simulink model "PEMFuelCellSystem_GasMixture_cEGR_RouteA_v2_v01"  (R2025b)
settings: Solver=VariableStepAuto  StartTime=0.0  StopTime=2500  RelTol=1e-3  AbsTol=1e-3
model workspace: external: MATLAB File E:\agentwork_pemfc_cEGR_0519\04_Simulink物理网络模型\01_模型\RouteA_GasMixture_Derived\PEMFuelCellSystemWithACustomLibraryParameters.m (data not in the file)
undefined symbols (not defined in the file): anode_tube_D, cathode_tube_D, cegr_valve_max_area, cegr_valve_open_min_area, comp_rpm_TLU, coolant_num_layers, coolant_num_passes, coolant_tube_D, coolant_w_channels, env_p, env_T, env_yH20, env_yO2, radiator_air_area_fins, radiator_air_area_primary, radiator_eta_fin, radiator_N_tubes, radiator_rho, radiator_t_wall, radiator_tube_H, radiator_W, routeA_air_pid_Ki, routeA_air_pid_Kp, routeA_anode_source_conditioner_nominal_flow_kg_s, routeA_cathode_source_conditioner_nominal_flow_kg_s, routeA_egr_control_Ki_area, routeA_egr_control_Kp_area, routeA_egr_target_input_mode_id, routeA_egr_valve_actuator_tau, routeA_egr_valve_area_direct, routeA_target_egr_ratio_comp_in, routeA_voltage_current_max_A, routeA_voltage_current_min_A, routeA_voltage_pi_Ki, routeA_voltage_pi_Kp, stack_area, stack_iL, stack_mea_rho, stack_num_cells, stack_num_channels, stack_t_gdl, stack_t_membrane, stack_w_channels, tank_p, tank_T, tank_yH2
libraries: FuelCell_lib x67, fl_lib x67, nesl_utility x56, slpidlib x5
(part 3 of 6)

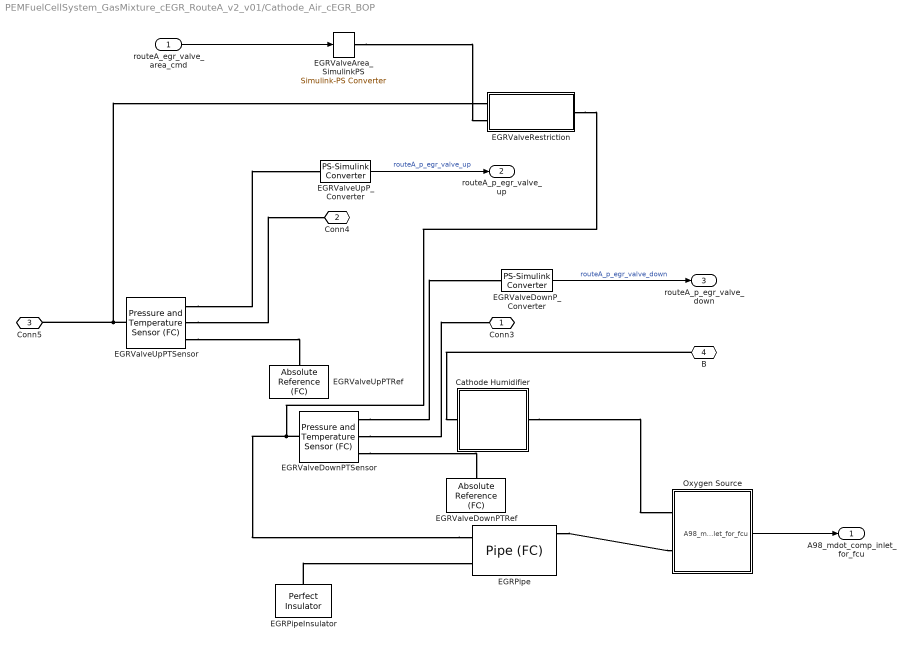
== system PEMFuelCellSystem_GasMixture_cEGR_RouteA_v2_v01/Cathode_Air_cEGR_BOP ==
  routeA_egr_valve_area_cmd : Inport
  Cathode Humidifier : Subsystem  Tag=PublishSubsystem
  EGRPipe : FuelCell_lib/elements/Pipe (FC)  length=cegr_pipe_length m  area=cegr_pipe_area m^2  Dh=cegr_pipe_D m  extra_length=cegr_pipe_extra_length m  roughness=cegr_pipe_roughness m  Re_lam=2000  Re_tur=4000  shape_factor=64  Nu_lam=3.66  tau_c=cegr_cond_tau s  isCond=[0; 0; 0; 1]  volMeas=false  compMeas=FuelCell.enum.Composition.Mole  p0=cegr_pipe_p0 MPa  T0=env_T degC  comp=FuelCell.enum.Composition.Mole  y0=[1-env_yO2-env_yH20; env_yO2; 0; env_yH20]  x0=[1-env_yO2-env_yH20; env_yO2; 0; env_yH20]
      settings: InternalSimscapePortConfiguration="{\"Bottom\":[{\"id\":\"MIn\",\"label\":\"M_in\",\"type\":\"input\"},{\"id\":\"TIn\",\"label\":\"T_in\",\"type\":\"input\"}],\"Left\":[{\"id\":\"A\",\"label\":\"A\",\"type\":\"FuelCell.FuelCell\"},{\"id\":\"H\",\"label\":\"H\",\"type\":\"foundation.thermal.thermal\"}],\"Right\":[{\"id\":\"B\",\"label\":\"B\",\"type\":\"FuelCell.FuelCell\"}],\"Top\":[]}"
  EGRPipeInsulator : fl_lib/Thermal/Thermal Elements/Perfect Insulator  T_specify=off  T_priority=None  T=293.15 K  T_nominal_specify=off  T_nominal_value=1  T_nominal_unit=K
  EGRValveArea_SimulinkPS : nesl_utility/Simulink-PS Converter  PhysicalDomain=network_engine_domain  SubClassName=ps_input  LeftPortType=input  RightPortType=output  PseudoPeriodic=off  Frequencies=[]  NoiseDistribution=none  NoiseParameters=[]  Unit=m^2  AffineConversion=off  FilteringAndDerivatives=provide  SimscapeFilterOrder=1  InputFilterTimeConstant=0.001  UdotUserProvided=0
  EGRValveDownPTRef : FuelCell_lib/elements/Absolute Reference (FC)
      settings: InternalSimscapePortConfiguration="{\"Bottom\":[],\"Left\":[{\"id\":\"A\",\"label\":\"\",\"type\":\"FuelCell.FuelCell\"}],\"Right\":[],\"Top\":[]}"
  EGRValveDownPTSensor : FuelCell_lib/sensors/Pressure and Temperature Sensor (FC)
      settings: InternalSimscapePortConfiguration="{\"Bottom\":[],\"Left\":[{\"id\":\"A\",\"label\":\"A\",\"type\":\"FuelCell.FuelCell\"}],\"Right\":[{\"id\":\"P\",\"label\":\"P\",\"type\":\"output\"},{\"id\":\"T\",\"label\":\"T\",\"type\":\"output\"},{\"id\":\"B\",\"label\":\"B\",\"type\":\"FuelCell.FuelCell\"}],\"Top\":[]}"
  EGRValveDownP_Converter : nesl_utility/PS-Simulink Converter  PhysicalDomain=network_engine_domain  SubClassName=ps_output  LeftPortType=input  RightPortType=output  PseudoPeriodic=off  Frequencies=[]  VectorFormat=inherit  Unit=inherit  AffineConversion=off
  EGRValveRestriction : Subsystem  Variant=on
  EGRValveUpPTRef : FuelCell_lib/elements/Absolute Reference (FC)
      settings: InternalSimscapePortConfiguration="{\"Bottom\":[],\"Left\":[{\"id\":\"A\",\"label\":\"\",\"type\":\"FuelCell.FuelCell\"}],\"Right\":[],\"Top\":[]}"
  EGRValveUpPTSensor : FuelCell_lib/sensors/Pressure and Temperature Sensor (FC)
      settings: InternalSimscapePortConfiguration="{\"Bottom\":[],\"Left\":[{\"id\":\"A\",\"label\":\"A\",\"type\":\"FuelCell.FuelCell\"}],\"Right\":[{\"id\":\"P\",\"label\":\"P\",\"type\":\"output\"},{\"id\":\"T\",\"label\":\"T\",\"type\":\"output\"},{\"id\":\"B\",\"label\":\"B\",\"type\":\"FuelCell.FuelCell\"}],\"Top\":[]}"
  EGRValveUpP_Converter : nesl_utility/PS-Simulink Converter  PhysicalDomain=network_engine_domain  SubClassName=ps_output  LeftPortType=input  RightPortType=output  PseudoPeriodic=off  Frequencies=[]  VectorFormat=inherit  Unit=inherit  AffineConversion=off
  Oxygen Source : Subsystem  Tag=PublishSubsystem
      mask Display:
      | plot(0, 0)
      | plot(100, 100)
      | 
      | n = 80;
      | r1 = 15;
      | r2 = 30;
      | 
      | plot(cos(linspace(0, 2*pi, n))*r1 + 65, sin(linspace(0, 2*pi, n))*r1 + 50)
      | plot(cos(linspace(0, 2*pi, n))*r2 + 65, sin(linspace(0, 2*pi, n))*r2 + 50)
      | 
      | plot([65 30 30 42], [80 80 70 70])
  Conn3 : PMIOPort  Side=Right
  Conn4 : PMIOPort  Port=2  Side=Right
  Conn5 : PMIOPort  Port=3  Side=Left
  B : PMIOPort  Port=4  Side=Left
  A98_mdot_comp_inlet_for_fcu : Outport
  routeA_p_egr_valve_up : Outport  Port=2
  routeA_p_egr_valve_down : Outport  Port=3
  wires:
  routeA_egr_valve_area_cmd/1 -> EGRValveArea_SimulinkPS/1
  EGRValveUpP_Converter/1 -> routeA_p_egr_valve_up/1  "routeA_p_egr_valve_up"
  EGRValveDownP_Converter/1 -> routeA_p_egr_valve_down/1  "routeA_p_egr_valve_down"
  Oxygen Source/1(A98_mdot_comp_inlet_for_fcu) -> A98_mdot_comp_inlet_for_fcu/1
  connections:
  EGRValveUpPTSensor/RConn2 -- Conn4/RConn1
  EGRValveUpPTSensor/RConn1 -- EGRValveUpP_Converter/LConn1
  EGRPipeInsulator/LConn1 -- EGRPipe/LConn2
  EGRValveDownPTSensor/RConn1 -- EGRValveDownP_Converter/LConn1
  EGRValveUpPTSensor/RConn3 -- EGRValveUpPTRef/LConn1
  EGRValveDownPTSensor/RConn2 -- Conn3/RConn1
  EGRValveDownPTSensor/RConn3 -- EGRValveDownPTRef/LConn1
  EGRPipe/RConn1 -- Oxygen Source/LConn2
  Cathode Humidifier/RConn1 -- Oxygen Source/LConn1
  B/RConn1 -- Cathode Humidifier/LConn1
  Conn5/RConn1 -- EGRValveUpPTSensor/LConn1 -- EGRValveRestriction/LConn1
  EGRPipe/LConn1 -- EGRValveDownPTSensor/LConn1 -- EGRValveRestriction/RConn1
  EGRValveArea_SimulinkPS/RConn1 -- EGRValveRestriction/LConn2

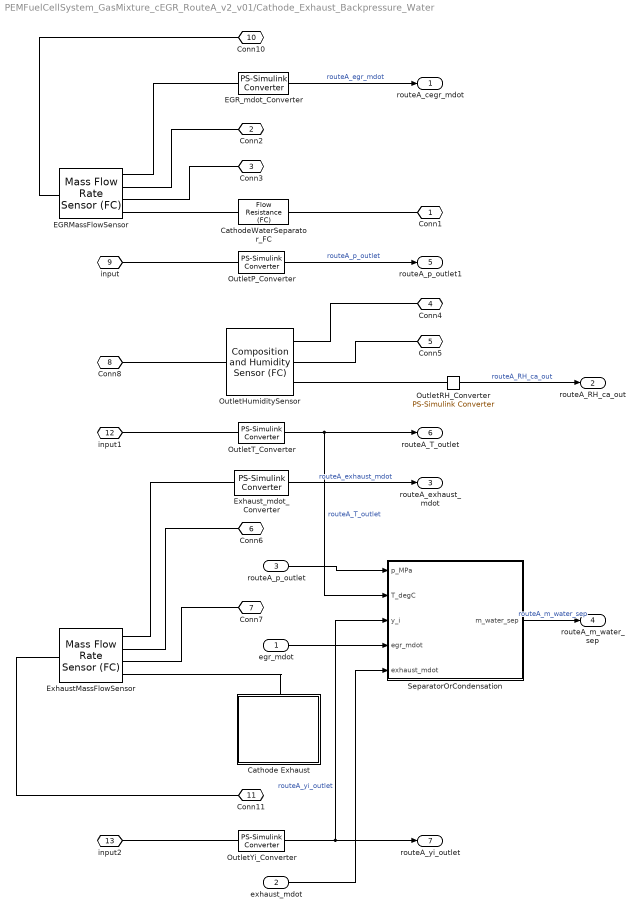
== system PEMFuelCellSystem_GasMixture_cEGR_RouteA_v2_v01/Cathode_Exhaust_Backpressure_Water ==
  egr_mdot : Inport
  exhaust_mdot : Inport  Port=2
  routeA_p_outlet : Inport  Port=3
  Cathode Exhaust : Subsystem  Tag=PublishSubsystem
      settings: PortSchema="{\"entries\":[{\"content\":{\"sides\":[{\"content\":{\"connectorIds\":[]},\"type\":\"ConnectorPlacement.EquallySpacedRectSide\",\"uuid\":\"6344d1cf-22ea-4a51-9588-07afca0fac15\"},{\"content\":{\"connectorIds\":[],\"side\":\"RIGHT\"},\"type\":\"ConnectorPlacement.EquallySpacedRectSide\",\"uuid\":\"a3908f81-9410-4056-87cd-9faba76d3fb8\"},{\"content\":{\"connectorIds\":[\"LConn1\"],\"side\":\"TOP\"},\"type\":\"ConnectorPlacement.EquallySpacedRectSide\",\"uuid\":\"a1c9e24d-adb9-4361-8e9b-feafccbbdb81\"}]},\"type\":\"ConnectorPlacement.EquallySpacedConnector\",\"uuid\":\"d5180d8f-18a0-491d-9fff-909db43c9aea\"}],\"packageUris\":[\"http://schema.mathworks.com/mf0/Connector/R2020b\"],\"version\":\"1.0\"}"
  CathodeWaterSeparator_FC : FuelCell_lib/elements/Flow Resistance (FC)  var_res=false  delta_p_nominal=cathode_separator_dp_nominal MPa  mdot_nominal=cathode_separator_mdot_nominal kg/s  rho_nominal=0 kg/m^3  laminar_fraction=cathode_separator_laminar_fraction  area=cathode_separator_area m^2  leak_thresh=1e-5
      settings: InternalSimscapePortConfiguration="{\"Bottom\":[],\"Left\":[{\"id\":\"A\",\"label\":\"A\",\"type\":\"FuelCell.FuelCell\"}],\"Right\":[{\"id\":\"B\",\"label\":\"B\",\"type\":\"FuelCell.FuelCell\"}],\"Top\":[]}"
  EGRMassFlowSensor : FuelCell_lib/sensors/Mass Flow Rate Sensor (FC)
      settings: InternalSimscapePortConfiguration="{\"Bottom\":[],\"Left\":[{\"id\":\"A\",\"label\":\"A\",\"type\":\"FuelCell.FuelCell\"}],\"Right\":[{\"id\":\"M\",\"label\":\"M\",\"type\":\"output\"},{\"id\":\"Phi_out\",\"label\":\"Phi\",\"type\":\"output\"},{\"id\":\"M_i\",\"label\":\"M_i\",\"type\":\"output\"},{\"id\":\"B\",\"label\":\"B\",\"type\":\"FuelCell.FuelCell\"}],\"Top\":[]}"
  EGR_mdot_Converter : nesl_utility/PS-Simulink Converter  PhysicalDomain=network_engine_domain  SubClassName=ps_output  LeftPortType=input  RightPortType=output  PseudoPeriodic=off  Frequencies=[]  VectorFormat=inherit  Unit=inherit  AffineConversion=off
  ExhaustMassFlowSensor : FuelCell_lib/sensors/Mass Flow Rate Sensor (FC)
      settings: InternalSimscapePortConfiguration="{\"Bottom\":[],\"Left\":[{\"id\":\"A\",\"label\":\"A\",\"type\":\"FuelCell.FuelCell\"}],\"Right\":[{\"id\":\"M\",\"label\":\"M\",\"type\":\"output\"},{\"id\":\"Phi_out\",\"label\":\"Phi\",\"type\":\"output\"},{\"id\":\"M_i\",\"label\":\"M_i\",\"type\":\"output\"},{\"id\":\"B\",\"label\":\"B\",\"type\":\"FuelCell.FuelCell\"}],\"Top\":[]}"
  Exhaust_mdot_Converter : nesl_utility/PS-Simulink Converter  PhysicalDomain=network_engine_domain  SubClassName=ps_output  LeftPortType=input  RightPortType=output  PseudoPeriodic=off  Frequencies=[]  VectorFormat=inherit  Unit=inherit  AffineConversion=off
  OutletHumiditySensor : FuelCell_lib/sensors/Composition and Humidity Sensor (FC)
      settings: InternalSimscapePortConfiguration="{\"Bottom\":[],\"Left\":[{\"id\":\"A\",\"label\":\"A\",\"type\":\"FuelCell.FuelCell\"}],\"Right\":[{\"id\":\"x_i\",\"label\":\"x_i\",\"type\":\"output\"},{\"id\":\"y_i\",\"label\":\"y_i\",\"type\":\"output\"},{\"id\":\"W\",\"label\":\"W\",\"type\":\"output\"}],\"Top\":[]}"
  OutletP_Converter : nesl_utility/PS-Simulink Converter  PhysicalDomain=network_engine_domain  SubClassName=ps_output  LeftPortType=input  RightPortType=output  PseudoPeriodic=off  Frequencies=[]  VectorFormat=inherit  Unit=inherit  AffineConversion=off
  OutletRH_Converter : nesl_utility/PS-Simulink Converter  PhysicalDomain=network_engine_domain  SubClassName=ps_output  LeftPortType=input  RightPortType=output  PseudoPeriodic=off  Frequencies=[]  VectorFormat=inherit  Unit=inherit  AffineConversion=off
  OutletT_Converter : nesl_utility/PS-Simulink Converter  PhysicalDomain=network_engine_domain  SubClassName=ps_output  LeftPortType=input  RightPortType=output  PseudoPeriodic=off  Frequencies=[]  VectorFormat=inherit  Unit=inherit  AffineConversion=off
  OutletYi_Converter : nesl_utility/PS-Simulink Converter  PhysicalDomain=network_engine_domain  SubClassName=ps_output  LeftPortType=input  RightPortType=output  PseudoPeriodic=off  Frequencies=[]  VectorFormat=inherit  Unit=inherit  AffineConversion=off
  SeparatorOrCondensation : MATLAB Function  Description=KPI observer only: estimates possible separated or condensed water from outlet p/T/y_i and branch mass flows. It is not the physical separator device.  TreatAsAtomicUnit=on
  Conn1 : PMIOPort  Side=Right
  Conn2 : PMIOPort  Port=2  Side=Right
  Conn3 : PMIOPort  Port=3  Side=Right
  Conn4 : PMIOPort  Port=4  Side=Right
  Conn5 : PMIOPort  Port=5  Side=Right
  Conn6 : PMIOPort  Port=6  Side=Right
  Conn7 : PMIOPort  Port=7  Side=Right
  Conn8 : PMIOPort  Port=8  Side=Left
  input : PMIOPort  Port=9  Side=Left
  Conn10 : PMIOPort  Port=10  Side=Left
  Conn11 : PMIOPort  Port=11  Side=Left
  input1 : PMIOPort  Port=12  Side=Left
  input2 : PMIOPort  Port=13  Side=Left
  routeA_cegr_mdot : Outport
  routeA_RH_ca_out : Outport  Port=2
  routeA_exhaust_mdot : Outport  Port=3
  routeA_m_water_sep : Outport  Port=4
  routeA_p_outlet1 : Outport  Port=5
  routeA_T_outlet : Outport  Port=6
  routeA_yi_outlet : Outport  Port=7
  wires:
  egr_mdot/1 -> SeparatorOrCondensation/4(egr_mdot)
  OutletT_Converter/1 -> routeA_T_outlet/1, SeparatorOrCondensation/2(T_degC)  "routeA_T_outlet"
  Exhaust_mdot_Converter/1 -> routeA_exhaust_mdot/1  "routeA_exhaust_mdot"
  EGR_mdot_Converter/1 -> routeA_cegr_mdot/1  "routeA_egr_mdot"
  OutletP_Converter/1 -> routeA_p_outlet1/1  "routeA_p_outlet"
  SeparatorOrCondensation/1(m_water_sep) -> routeA_m_water_sep/1  "routeA_m_water_sep"
  routeA_p_outlet/1 -> SeparatorOrCondensation/1(p_MPa)
  OutletYi_Converter/1 -> SeparatorOrCondensation/3(y_i), routeA_yi_outlet/1  "routeA_yi_outlet"
  exhaust_mdot/1 -> SeparatorOrCondensation/5(exhaust_mdot)
  OutletRH_Converter/1 -> routeA_RH_ca_out/1  "routeA_RH_ca_out"
  connections:
  input1/RConn1 -- OutletT_Converter/LConn1
  Conn8/RConn1 -- OutletHumiditySensor/LConn1
  EGRMassFlowSensor/RConn1 -- EGR_mdot_Converter/LConn1
  ExhaustMassFlowSensor/RConn1 -- Exhaust_mdot_Converter/LConn1
  EGRMassFlowSensor/RConn2 -- Conn2/RConn1
  EGRMassFlowSensor/RConn3 -- Conn3/RConn1
  input/RConn1 -- OutletP_Converter/LConn1
  EGRMassFlowSensor/RConn4 -- CathodeWaterSeparator_FC/LConn1
  ExhaustMassFlowSensor/RConn2 -- Conn6/RConn1
  ExhaustMassFlowSensor/RConn3 -- Conn7/RConn1
  ExhaustMassFlowSensor/RConn4 -- Cathode Exhaust/LConn1
  input2/RConn1 -- OutletYi_Converter/LConn1
  Conn10/RConn1 -- EGRMassFlowSensor/LConn1
  Conn11/RConn1 -- ExhaustMassFlowSensor/LConn1
  CathodeWaterSeparator_FC/RConn1 -- Conn1/RConn1
  OutletHumiditySensor/RConn1 -- Conn4/RConn1
  OutletHumiditySensor/RConn2 -- Conn5/RConn1
  OutletHumiditySensor/RConn3 -- OutletRH_Converter/LConn1

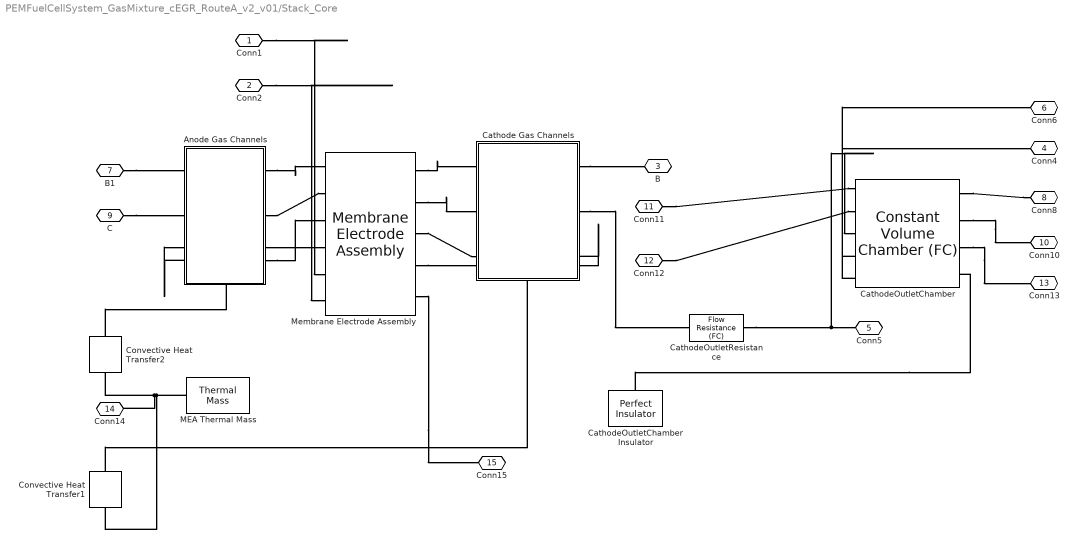
== system PEMFuelCellSystem_GasMixture_cEGR_RouteA_v2_v01/Stack_Core ==
  Anode Gas Channels : Subsystem  Tag=PublishSubsystem
      settings: PortSchema="{\"entries\":[{\"content\":{\"sides\":[{\"content\":{\"connectorIds\":[\"LConn1\",\"LConn2\",\"LConn3\"]},\"type\":\"ConnectorPlacement.EquallySpacedRectSide\",\"uuid\":\"f0c92738-2de1-40ac-9e4a-670524600aa2\"},{\"content\":{\"connectorIds\":[\"RConn1\",\"RConn2\",\"RConn3\"],\"side\":\"RIGHT\"},\"type\":\"ConnectorPlacement.EquallySpacedRectSide\",\"uuid\":\"f0ed995d-2dce-4bd6-9faa-b1cb502a30b1\"},{\"content\":{\"connectorIds\":[],\"side\":\"TOP\"},\"type\":\"ConnectorPlacement.EquallySpacedRectSide\",\"uuid\":\"b5d2d698-46b6-42b5-a767-bb9f1790aa28\"},{\"content\":{\"connectorIds\":[\"RConn4\"],\"side\":\"BOTTOM\"},\"type\":\"ConnectorPlacement.EquallySpacedRectSide\",\"uuid\":\"3e8c99a3-0044-43a9-bacb-b652445e4ac6\"}]},\"type\":\"ConnectorPlacement.EquallySpacedConnector\",\"uuid\":\"912925fb-ca80-4fe6-8a1d-a2308cfd6f88\"}],\"packageUris\":[\"http://schema.mathworks.com/mf0/Connector/R2020b\"],\"version\":\"1.0\"}"
      mask Display:
      | plot(0, 0)
      | plot(100, 100)
      | 
      | x1 = 25;
      | x2 = 65;
      | y1 = 23;
      | y2 = 95;
      | xt = 15;
      | yt = 9;
      | 
      | x_pattern = [x2 x2    x1+xt x1+xt   x1+xt   x2     ];
      | y_pattern = [y2 y2-yt y2-yt y2-2*yt y2-2*yt y2-2*yt];
      | 
      | plot([x1 x1 x2 x_pattern x_pattern      x_pattern      x_pattern         x2    x1], ...
      |      [y1-yt y2 y2 y_pattern y_pattern-2*yt y_pattern-4*yt y_pattern-6*yt y1-yt y1-yt])
  Cathode Gas Channels : Subsystem  Tag=PublishSubsystem
      settings: PortSchema="{\"entries\":[{\"content\":{\"sides\":[{\"content\":{\"connectorIds\":[\"LConn1\",\"LConn2\",\"LConn3\"]},\"type\":\"ConnectorPlacement.EquallySpacedRectSide\",\"uuid\":\"f0c92738-2de1-40ac-9e4a-670524600aa2\"},{\"content\":{\"connectorIds\":[\"RConn1\",\"RConn2\",\"RConn3\"],\"side\":\"RIGHT\"},\"type\":\"ConnectorPlacement.EquallySpacedRectSide\",\"uuid\":\"f0ed995d-2dce-4bd6-9faa-b1cb502a30b1\"},{\"content\":{\"connectorIds\":[],\"side\":\"TOP\"},\"type\":\"ConnectorPlacement.EquallySpacedRectSide\",\"uuid\":\"b5d2d698-46b6-42b5-a767-bb9f1790aa28\"},{\"content\":{\"connectorIds\":[\"RConn4\"],\"side\":\"BOTTOM\"},\"type\":\"ConnectorPlacement.EquallySpacedRectSide\",\"uuid\":\"3e8c99a3-0044-43a9-bacb-b652445e4ac6\"}]},\"type\":\"ConnectorPlacement.EquallySpacedConnector\",\"uuid\":\"912925fb-ca80-4fe6-8a1d-a2308cfd6f88\"}],\"packageUris\":[\"http://schema.mathworks.com/mf0/Connector/R2020b\"],\"version\":\"1.0\"}"
      mask Display:
      | plot(0, 0)
      | plot(100, 100)
      | 
      | x1 = 25;
      | x2 = 65;
      | y1 = 23;
      | y2 = 95;
      | xt = 15;
      | yt = 9;
      | 
      | x_pattern = [x2 x2    x1+xt x1+xt   x1+xt   x2     ];
      | y_pattern = [y2 y2-yt y2-yt y2-2*yt y2-2*yt y2-2*yt];
      | 
      | plot([x1 x1 x2 x_pattern x_pattern      x_pattern      x_pattern         x2    x1], ...
      |      [y1-yt y2 y2 y_pattern y_pattern-2*yt y_pattern-4*yt y_pattern-6*yt y1-yt y1-yt])
  CathodeOutletChamber : FuelCell_lib/elements/Constant Volume Chamber (FC)  V0=cathode_outlet_chamber_V l  num_ports=foundation.enum.num_ports.three  area_A=cegr_pipe_area m^2  area_B=cegr_pipe_area m^2  area_C=cegr_pipe_area m^2  area_D=0.01 m^2  cond_spec=FuelCell.enum.ChamberCondSpec.Enabled  tau_c=cegr_cond_tau s  is_cond=[0; 0; 0; 1]  out_comp=FuelCell.enum.Composition.Mole  p0=cegr_outlet_chamber_p0 MPa  T0=env_T degC  comp=FuelCell.enum.Composition.Mole  y0=[1-env_yO2-env_yH20; env_yO2; 0; env_yH20]  x0=[1-env_yO2-env_yH20; env_yO2; 0; env_yH20]
      settings: InternalSimscapePortConfiguration="{\"Bottom\":[{\"id\":\"H\",\"label\":\"H\",\"type\":\"foundation.thermal.thermal\"}],\"Left\":[{\"id\":\"MIn\",\"label\":\"MIn\",\"type\":\"input\"},{\"id\":\"TIn\",\"label\":\"TIn\",\"type\":\"input\"}],\"Right\":[{\"id\":\"pC\",\"label\":\"p\",\"type\":\"output\"},{\"id\":\"TC\",\"label\":\"T\",\"type\":\"output\"},{\"id\":\"yC_i\",\"label\":\"y_i\",\"type\":\"output\"}],\"Top\":[{\"id\":\"A\",\"label\":\"A\",\"type\":\"FuelCell.FuelCell\"},{\"id\":\"B\",\"label\":\"B\",\"type\":\"FuelCell.FuelCell\"},{\"id\":\"C\",\"label\":\"C\",\"type\":\"FuelCell.FuelCell\"}]}"
  CathodeOutletChamberInsulator : fl_lib/Thermal/Thermal Elements/Perfect Insulator  T_specify=off  T_priority=None  T=293.15 K  T_nominal_specify=off  T_nominal_value=1  T_nominal_unit=K
  CathodeOutletResistance : FuelCell_lib/elements/Flow Resistance (FC)  var_res=false  delta_p_nominal=0.001 MPa  mdot_nominal=0.1 kg/s  rho_nominal=0 kg/m^3  laminar_fraction=1e-3  area=cegr_pipe_area m^2  leak_thresh=1e-5
      settings: InternalSimscapePortConfiguration="{\"Bottom\":[],\"Left\":[{\"id\":\"A\",\"label\":\"A\",\"type\":\"FuelCell.FuelCell\"}],\"Right\":[{\"id\":\"B\",\"label\":\"B\",\"type\":\"FuelCell.FuelCell\"}],\"Top\":[]}"
  Convective Heat Transfer1 : fl_lib/Thermal/Thermal Elements/Convective Heat Transfer  thermal_type=foundation.enum.constant_variable.constant  area=stack_w_channels^2 * stack_num_channels * stack_num_cells cm^2  heat_tr_coeff=10 W/(m^2 * K)  min_heat_tr_coeff=1e-3 W/(K*m^2)  T_specify=off  T_priority=None  T=0 K  T_nominal_specify=off  T_nominal_value=1  T_nominal_unit=K  Q_specify=off  Q_priority=None  Q=0 W  Q_nominal_specify=off  Q_nominal_value=1  Q_nominal_unit=W
  Convective Heat Transfer2 : fl_lib/Thermal/Thermal Elements/Convective Heat Transfer  thermal_type=foundation.enum.constant_variable.constant  area=stack_w_channels^2 * stack_num_channels * stack_num_cells cm^2  heat_tr_coeff=10 W/(m^2 * K)  min_heat_tr_coeff=1e-3 W/(K*m^2)  T_specify=off  T_priority=None  T=0 K  T_nominal_specify=off  T_nominal_value=1  T_nominal_unit=K  Q_specify=off  Q_priority=None  Q=0 W  Q_nominal_specify=off  Q_nominal_value=1  Q_nominal_unit=W
  MEA Thermal Mass : fl_lib/Thermal/Thermal Elements/Thermal Mass  mass_type=foundation.enum.constant_variable.constant  mass=stack_mea_rho * stack_area*1e-4 * (stack_t_membrane + 2*stack_t_gdl)*1e-6 * stack_num_cells kg  sp_heat=stack_mea_cp J/kg/K  mass_min=1e-6 kg  num_ports=foundation.enum.numPorts2.one  m_specify=off  m_priority=High  m=1 kg  m_nominal_specify=off  m_nominal_value=1  m_nominal_unit=kg  T_specify=on  T_priority=High  T=env_T degC  T_nominal_specify=off  T_nominal_value=1  T_nominal_unit=K  Q_specify=off  Q_priority=None  Q=0 W  Q_nominal_specify=off  Q_nominal_value=1  Q_nominal_unit=W
  Membrane Electrode Assembly : FuelCell_lib/elements/Membrane Electrode Assembly  N_cell=stack_num_cells  area_cell=stack_area cm^2  t_membrane=stack_t_membrane um  rtype=FuelCell.enum.ResistanceModel.Tabulated1D  RH_TLU=[0, .1, .2, .3, .4, .5, .6, .7, .8, .9, 1]  conductivity_TLU_1D=[0, .017, .035, .055, .081, .11, .15, .21, .27, .35, .45] S/cm  T_scale=1268 K  T_cond=353.15 K  T_TLU=[303.15, 353.15, 393.15] K  conductivity_TLU_2D=[0, .0093, .019, .031, .045, .063, .086, .11, .15, .2, .25; 0, .017, .035, .055, .081, .11, .15, .21, .27, .35, .45; 0, .024, .05, .08, .12, .16, .22, .3, .39, .51, .65] S/cm  io=stack_io A/cm^2  iL=stack_iL A/cm^2  alpha=stack_alpha  rho_membrane=2000 kg/m^3  M_membrane=1.1 kg/mol  D_N2=1e-5 cm^2/s  Icell_specify=off  Icell_priority=None  Icell=0 A  Icell_nominal_specify=off  Icell_nominal_value=1  Icell_nominal_unit=A  HeatRxn_specify=off  HeatRxn_priority=None  HeatRxn=0 W  HeatRxn_nominal_specify=off  HeatRxn_nominal_value=1  HeatRxn_nominal_unit=W  T_stack_specify=off  T_stack_priority=None  T_stack=353.15 K  T_stack_nominal_specify=off  T_stack_nominal_value=1  T_stack_nominal_unit=K
      settings: InternalSimscapePortConfiguration="{\"Bottom\":[{\"id\":\"H\",\"label\":\"H\",\"type\":\"foundation.thermal.thermal\"}],\"Left\":[{\"id\":\"A\",\"label\":\"A\",\"type\":\"FuelCell.FuelCell\"},{\"id\":\"mdot_an\",\"label\":\"Ma\",\"type\":\"output\"},{\"id\":\"T_an\",\"label\":\"Ta\",\"type\":\"output\"},{\"id\":\"x_i_anode\",\"label\":\"xia\",\"type\":\"input\"}],\"Right\":[{\"id\":\"C\",\"label\":\"C\",\"type\":\"FuelCell.FuelCell\"},{\"id\":\"mdot_ca\",\"label\":\"Mc\",\"type\":\"output\"},{\"id\":\"T_ca\",\"label\":\"Tc\",\"type\":\"output\"},{\"id\":\"x_i_cathode\",\"label\":\"xic\",\"type\":\"input\"}],\"Top\":[{\"id\":\"n\",\"label\":\"-\",\"type\":\"foundation.electrical.electrical\"},{\"id\":\"p\",\"label\":\"+\",\"type\":\"foundation.electrical.electrical\"}]}"
  Conn1 : PMIOPort  Side=Left
  Conn2 : PMIOPort  Port=2  Side=Left
  B : PMIOPort  Port=3  Side=Left
  Conn4 : PMIOPort  Port=4  Side=Left
  Conn5 : PMIOPort  Port=5  Side=Right
  Conn6 : PMIOPort  Port=6  Side=Left
  B1 : PMIOPort  Port=7  Side=Left
  Conn8 : PMIOPort  Port=8  Side=Right
  C : PMIOPort  Port=9  Side=Left
  Conn10 : PMIOPort  Port=10  Side=Right
  Conn11 : PMIOPort  Port=11  Side=Left
  Conn12 : PMIOPort  Port=12  Side=Left
  Conn13 : PMIOPort  Port=13  Side=Right
  Conn14 : PMIOPort  Port=14  Side=Left
  Conn15 : PMIOPort  Port=15  Side=Right
  connections:
  B1/RConn1 -- Anode Gas Channels/LConn1
  C/RConn1 -- Anode Gas Channels/LConn2
  Convective Heat Transfer2/LConn1 -- Anode Gas Channels/RConn4
  Conn1/RConn1 -- Membrane Electrode Assembly/LConn5
  MEA Thermal Mass/LConn1 -- Convective Heat Transfer2/RConn1 -- Conn14/RConn1 -- Convective Heat Transfer1/RConn1
  Conn2/RConn1 -- Membrane Electrode Assembly/LConn6
  Convective Heat Transfer1/LConn1 -- Cathode Gas Channels/RConn4
  Anode Gas Channels/LConn3 -- Membrane Electrode Assembly/LConn4
  Membrane Electrode Assembly/RConn4 -- Cathode Gas Channels/LConn3
  Anode Gas Channels/RConn1 -- Membrane Electrode Assembly/LConn1
  Anode Gas Channels/RConn2 -- Membrane Electrode Assembly/LConn2
  Anode Gas Channels/RConn3 -- Membrane Electrode Assembly/LConn3
  Membrane Electrode Assembly/RConn5 -- Conn15/RConn1
  Membrane Electrode Assembly/RConn2 -- Cathode Gas Channels/RConn2
  Membrane Electrode Assembly/RConn1 -- Cathode Gas Channels/RConn1
  Membrane Electrode Assembly/RConn3 -- Cathode Gas Channels/RConn3
  Cathode Gas Channels/LConn1 -- B/RConn1
  Cathode Gas Channels/LConn2 -- CathodeOutletResistance/LConn1
  Conn11/RConn1 -- CathodeOutletChamber/LConn1
  Conn12/RConn1 -- CathodeOutletChamber/LConn2
  CathodeOutletResistance/RConn1 -- Conn5/RConn1 -- CathodeOutletChamber/LConn3
  CathodeOutletChamberInsulator/LConn1 -- CathodeOutletChamber/RConn4
  CathodeOutletChamber/RConn2 -- Conn10/RConn1
  CathodeOutletChamber/RConn1 -- Conn8/RConn1
  CathodeOutletChamber/LConn5 -- Conn4/RConn1
  CathodeOutletChamber/RConn3 -- Conn13/RConn1
  CathodeOutletChamber/LConn4 -- Conn6/RConn1

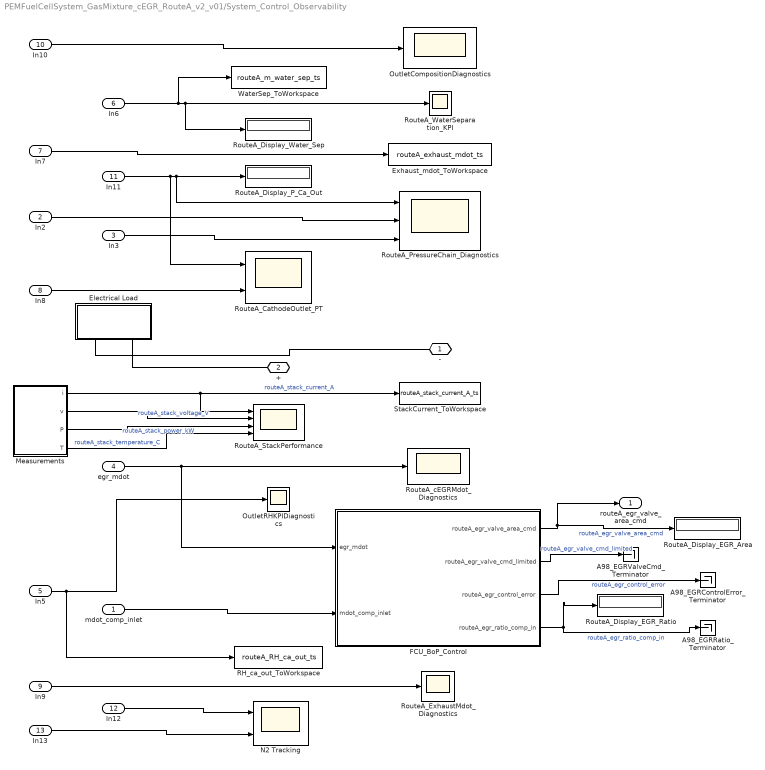
== system PEMFuelCellSystem_GasMixture_cEGR_RouteA_v2_v01/System_Control_Observability ==
  mdot_comp_inlet : Inport
  In2 : Inport  Port=2
  In3 : Inport  Port=3
  egr_mdot : Inport  Port=4
  In5 : Inport  Port=5
  In6 : Inport  Port=6
  In7 : Inport  Port=7
  In8 : Inport  Port=8
  In9 : Inport  Port=9
  In10 : Inport  Port=10
  In11 : Inport  Port=11
  In12 : Inport  Port=12
  In13 : Inport  Port=13
  A98_EGRControlError_Terminator : Terminator
  A98_EGRRatio_Terminator : Terminator
  A98_EGRValveCmd_Terminator : Terminator
  Electrical Load : Subsystem  Tag=PublishSubsystem  mask(Electrical Load){input_type=Current}
      mask prompts: input_type "Select one of the following scenarios:"
      settings: PortSchema="{\"entries\":[{\"content\":{\"sides\":[{\"content\":{\"connectorIds\":[]},\"type\":\"ConnectorPlacement.EquallySpacedRectSide\",\"uuid\":\"cf26c57a-4aaa-4eca-a1cf-dab3379228b7\"},{\"content\":{\"connectorIds\":[],\"side\":\"RIGHT\"},\"type\":\"ConnectorPlacement.EquallySpacedRectSide\",\"uuid\":\"bd4a28c6-f8d3-4492-9f61-a12eb17ccdd3\"},{\"content\":{\"connectorIds\":[],\"side\":\"TOP\"},\"type\":\"ConnectorPlacement.EquallySpacedRectSide\",\"uuid\":\"7f54a4db-ccf4-4e3a-a135-4ada067d241f\"},{\"content\":{\"connectorIds\":[\"RConn1\",\"RConn2\"],\"side\":\"BOTTOM\"},\"type\":\"ConnectorPlacement.EquallySpacedRectSide\",\"uuid\":\"8817983d-3f79-43b3-9594-6d12f7dcf066\"}]},\"type\":\"ConnectorPlacement.EquallySpacedConnector\",\"uuid\":\"79253ea6-cd7f-4983-840a-f5cee3a4dd91\"}],\"packageUris\":[\"http://schema.mathworks.com/mf0/Connector/R2020b\"],\"version\":\"1.0\"}"
      mask TypeOptions input_type: Current | Power | Voltage
      mask Callback input_type:
      | activeVariant = get_param(gcb, 'input_type');
      | set_param([gcb '/Inputs'], 'OverrideUsingVariant', activeVariant)
      mask Display:
      | blk = get_param([gcb, '/Inputs'], 'CompiledActiveChoiceBlock');
      | eval(get_param(blk, 'MaskDisplay'))
  Exhaust_mdot_ToWorkspace : ToWorkspace  VariableName=routeA_exhaust_mdot_ts  SaveFormat=Timeseries  SampleTime=-1
  FCU_BoP_Control : Subsystem
  Measurements : Subsystem
  N2 Tracking : Scope  NumInputPorts=2
      settings: Title=Anode Nitrogen Molar Fraction and Purge Valve Activation  ActiveDisplayYMinimum=-0.125  ActiveDisplayYMaximum=1.125
  OutletCompositionDiagnostics : Scope
  OutletRHKPIDiagnostics : Scope
  RH_ca_out_ToWorkspace : ToWorkspace  VariableName=routeA_RH_ca_out_ts  SaveFormat=Timeseries
  RouteA_CathodeOutlet_PT : Scope  NumInputPorts=2
  RouteA_Display_EGR_Area : Display
  RouteA_Display_EGR_Ratio : Display
  RouteA_Display_P_Ca_Out : Display
  RouteA_Display_Water_Sep : Display
  RouteA_ExhaustMdot_Diagnostics : Scope
  RouteA_PressureChain_Diagnostics : Scope  NumInputPorts=3
  RouteA_StackPerformance : Scope  NumInputPorts=4
      settings: Title=Current (A)  ActiveDisplayYMinimum=-30.6721  ActiveDisplayYMaximum=276.0489
  RouteA_WaterSeparation_KPI : Scope
  RouteA_cEGRMdot_Diagnostics : Scope
  StackCurrent_ToWorkspace : ToWorkspace  VariableName=routeA_stack_current_A_ts  SaveFormat=Timeseries
  WaterSep_ToWorkspace : ToWorkspace  VariableName=routeA_m_water_sep_ts  SaveFormat=Timeseries
  - : PMIOPort  Side=Right
  + : PMIOPort  Port=2  Side=Right
  routeA_egr_valve_area_cmd : Outport
  wires:
  FCU_BoP_Control/1(routeA_egr_valve_area_cmd) -> RouteA_Display_EGR_Area/1, routeA_egr_valve_area_cmd/1  "routeA_egr_valve_area_cmd"
  FCU_BoP_Control/2(routeA_egr_valve_cmd_limited) -> A98_EGRValveCmd_Terminator/1  "routeA_egr_valve_cmd_limited"
  FCU_BoP_Control/3(routeA_egr_control_error) -> A98_EGRControlError_Terminator/1  "routeA_egr_control_error"
  FCU_BoP_Control/4(routeA_egr_ratio_comp_in) -> RouteA_Display_EGR_Ratio/1, A98_EGRRatio_Terminator/1  "routeA_egr_ratio_comp_in"
  In12/1 -> N2 Tracking/1
  In13/1 -> N2 Tracking/2
  In9/1 -> RouteA_ExhaustMdot_Diagnostics/1
  mdot_comp_inlet/1 -> FCU_BoP_Control/2(mdot_comp_inlet)
  Measurements/1(i) -> StackCurrent_ToWorkspace/1, RouteA_StackPerformance/1  "routeA_stack_current_A"
  In8/1 -> RouteA_CathodeOutlet_PT/2
  egr_mdot/1 -> RouteA_cEGRMdot_Diagnostics/1, FCU_BoP_Control/1(egr_mdot)
  In5/1 -> OutletRHKPIDiagnostics/1, RH_ca_out_ToWorkspace/1
  In11/1 -> RouteA_PressureChain_Diagnostics/1, RouteA_Display_P_Ca_Out/1, RouteA_CathodeOutlet_PT/1
  In7/1 -> Exhaust_mdot_ToWorkspace/1
  Measurements/2(v) -> RouteA_StackPerformance/2  "routeA_stack_voltage_V"
  Measurements/3(P) -> RouteA_StackPerformance/3  "routeA_stack_power_kW"
  Measurements/4(T) -> RouteA_StackPerformance/4  "routeA_stack_temperature_C"
  In10/1 -> OutletCompositionDiagnostics/1
  In3/1 -> RouteA_PressureChain_Diagnostics/3
  In2/1 -> RouteA_PressureChain_Diagnostics/2
  In6/1 -> RouteA_Display_Water_Sep/1, RouteA_WaterSeparation_KPI/1, WaterSep_ToWorkspace/1
  connections:
  Electrical Load/RConn1 -- -/RConn1
  Electrical Load/RConn2 -- +/RConn1

== system PEMFuelCellSystem_GasMixture_cEGR_RouteA_v2_v01/Thermal_Management_BOP ==
  Cooling System : Subsystem  Tag=PublishSubsystem
      mask Display:
      | plot(0, 0)
      | plot(100, 100)
      | 
      | n = 80;
      | r = 35;
      | 
      | x = 45;
      | y = 50;
      | t = 5;
      | 
      | plot(cos(linspace(0, 2*pi, n))*r + x, sin(linspace(0, 2*pi, n))*r + y)
      | 
      | plot([x x x-r+t x+r-t x x], [y+r+2*t y+r-t y y y-r+t y-r-2*t])
  Heat Dissipation : Subsystem
      settings: PortSchema="{\"entries\":[{\"content\":{\"sides\":[{\"content\":{\"connectorIds\":[]},\"type\":\"ConnectorPlacement.EquallySpacedRectSide\",\"uuid\":\"40b2385a-b20e-464f-8016-3228e4acac4a\"},{\"content\":{\"connectorIds\":[],\"side\":\"RIGHT\"},\"type\":\"ConnectorPlacement.EquallySpacedRectSide\",\"uuid\":\"0e95dc4b-d2da-4ab6-a6e9-e2cb275776ce\"},{\"content\":{\"connectorIds\":[\"LConn1\"],\"side\":\"TOP\"},\"type\":\"ConnectorPlacement.EquallySpacedRectSide\",\"uuid\":\"0f5995c7-26f6-433d-889b-dea78bcd2b2a\"},{\"content\":{\"connectorIds\":[\"RConn1\"],\"side\":\"BOTTOM\"},\"type\":\"ConnectorPlacement.EquallySpacedRectSide\",\"uuid\":\"a2ee1c19-f9e9-4dbd-a9ff-92feea387e85\"}]},\"type\":\"ConnectorPlacement.EquallySpacedConnector\",\"uuid\":\"721753ea-9ada-4c74-8c6f-50b905d96904\"}],\"packageUris\":[\"http://schema.mathworks.com/mf0/Connector/R2020b\"],\"version\":\"1.0\"}"
  A : PMIOPort  Side=Left
  H : PMIOPort  Port=2  Side=Right
  connections:
  Heat Dissipation/RConn1 -- H/RConn1 -- Cooling System/RConn1
  Heat Dissipation/LConn1 -- A/RConn1

== system PEMFuelCellSystem_GasMixture_cEGR_RouteA_v2_v01/cEGR_Mode_Selector ==
  note: 1) Add Subsystem or Model blocks as valid variant choices.
      | 2) You cannot connect blocks at this level. At simulation, connectivity is automatically
      | determined, based on the active variant and port name matching.
  noCEGR_Isolation : Subsystem  VariantControl=routeA_cegr_enabled == 0
  withCEGR_PassThrough : Subsystem  VariantControl=routeA_cegr_enabled == 1
  A : PMIOPort  Side=Left
  B : PMIOPort  Port=2  Side=Left

== system PEMFuelCellSystem_GasMixture_cEGR_RouteA_v2_v01/Anode_Hydrogen_BOP/Anode Humidifier ==
  Composition and Humidity Sensor (FC) : FuelCell_lib/sensors/Composition and Humidity Sensor (FC)
      settings: InternalSimscapePortConfiguration="{\"Bottom\":[],\"Left\":[{\"id\":\"A\",\"label\":\"A\",\"type\":\"FuelCell.FuelCell\"}],\"Right\":[{\"id\":\"x_i\",\"label\":\"x_i\",\"type\":\"output\"},{\"id\":\"y_i\",\"label\":\"y_i\",\"type\":\"output\"},{\"id\":\"W\",\"label\":\"W\",\"type\":\"output\"}],\"Top\":[]}"
  PS Gain : fl_lib/Physical Signals/Functions/PS Gain  gain=[0;0;0;1]
  PS-Simulink Converter : nesl_utility/PS-Simulink Converter  PhysicalDomain=network_engine_domain  SubClassName=ps_output  LeftPortType=input  RightPortType=output  PseudoPeriodic=off  Frequencies=[]  VectorFormat=1-D array  Unit=1  AffineConversion=off
  Perfect Insulator : fl_lib/Thermal/Thermal Elements/Perfect Insulator  T_specify=off  T_priority=None  T=0 K  T_nominal_specify=off  T_nominal_value=1  T_nominal_unit=K
  Pipe (N Gas) : FuelCell_lib/elements/Pipe (FC)  length=0.25 m  area=pi*0.05^2/4 m^2  Dh=0.05 m  extra_length=0.1 m  roughness=15e-6 m  Re_lam=2000  Re_tur=4000  shape_factor=64  Nu_lam=3.66  tau_c=1e-3 s  isCond=[0; 0; 0; 0]  volMeas=false  compMeas=FuelCell.enum.Composition.Mole  p0=env_p MPa  T0=env_T degC  comp=FuelCell.enum.Composition.Mole  y0=[0; 0; 1; 0]  x0=[1; 0; 0; 0]
      settings: InternalSimscapePortConfiguration="{\"Bottom\":[{\"id\":\"MIn\",\"label\":\"M_in\",\"type\":\"input\"},{\"id\":\"TIn\",\"label\":\"T_in\",\"type\":\"input\"}],\"Left\":[{\"id\":\"A\",\"label\":\"A\",\"type\":\"FuelCell.FuelCell\"},{\"id\":\"H\",\"label\":\"H\",\"type\":\"foundation.thermal.thermal\"}],\"Right\":[{\"id\":\"B\",\"label\":\"B\",\"type\":\"FuelCell.FuelCell\"}],\"Top\":[]}"
  Proportional Control : Subsystem
  Simulink-PS Converter : nesl_utility/Simulink-PS Converter  PhysicalDomain=network_engine_domain  SubClassName=ps_input  LeftPortType=input  RightPortType=output  PseudoPeriodic=off  Frequencies=[]  NoiseDistribution=none  NoiseParameters=[]  Unit=kg/s  AffineConversion=off  FilteringAndDerivatives=provide  SimscapeFilterOrder=1  InputFilterTimeConstant=0.001  UdotUserProvided=0
  Simulink-PS Converter1 : nesl_utility/Simulink-PS Converter  PhysicalDomain=network_engine_domain  SubClassName=ps_input  LeftPortType=input  RightPortType=output  PseudoPeriodic=off  Frequencies=[]  NoiseDistribution=none  NoiseParameters=[]  Unit=degC  AffineConversion=on  FilteringAndDerivatives=provide  SimscapeFilterOrder=1  InputFilterTimeConstant=0.001  UdotUserProvided=0
  Transfer Fcn : TransferFcn  Denominator=[1 1]
  A : PMIOPort  Side=Left
  B : PMIOPort  Port=2  Side=Right
  wires:
  Transfer Fcn/1 -> Simulink-PS Converter1/1
  [T_stack] -> Transfer Fcn/1
  PS-Simulink Converter/1 -> Proportional Control/2(RH_meas)
  Proportional Control/1(Mw) -> Simulink-PS Converter/1
  [RouteA_CMD_anode_humidifier_rh] -> Proportional Control/1(RH_set)
  connections:
  PS Gain/LConn1 -- Simulink-PS Converter/RConn1
  Simulink-PS Converter1/RConn1 -- Pipe (N Gas)/RConn3
  PS-Simulink Converter/LConn1 -- Composition and Humidity Sensor (FC)/RConn3
  Pipe (N Gas)/RConn1 -- Composition and Humidity Sensor (FC)/LConn1 -- B/RConn1
  A/RConn1 -- Pipe (N Gas)/LConn1
  Perfect Insulator/LConn1 -- Pipe (N Gas)/LConn2
  PS Gain/RConn1 -- Pipe (N Gas)/RConn2

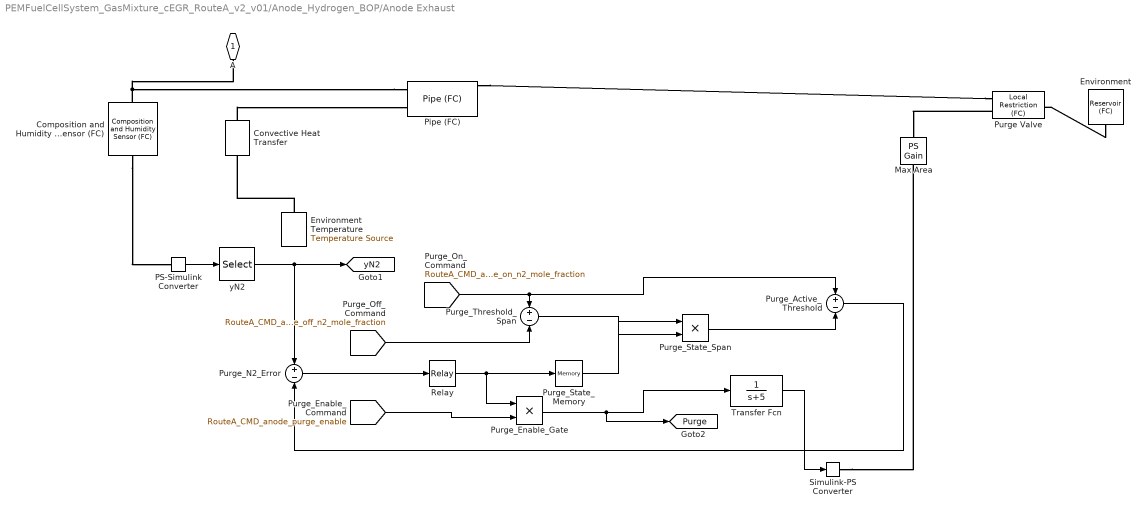
== system PEMFuelCellSystem_GasMixture_cEGR_RouteA_v2_v01/Anode_Hydrogen_BOP/Anode Exhaust ==
  Composition and Humidity Sensor (FC) : FuelCell_lib/sensors/Composition and Humidity Sensor (FC)
      settings: InternalSimscapePortConfiguration="{\"Bottom\":[],\"Left\":[{\"id\":\"A\",\"label\":\"A\",\"type\":\"FuelCell.FuelCell\"}],\"Right\":[{\"id\":\"x_i\",\"label\":\"x_i\",\"type\":\"output\"},{\"id\":\"y_i\",\"label\":\"y_i\",\"type\":\"output\"},{\"id\":\"W\",\"label\":\"W\",\"type\":\"output\"}],\"Top\":[]}"
  Convective Heat Transfer : fl_lib/Thermal/Thermal Elements/Convective Heat Transfer  thermal_type=foundation.enum.constant_variable.constant  area=pi*anode_tube_D^2/4 m^2  heat_tr_coeff=20 W/(m^2 * K)  min_heat_tr_coeff=1e-3 W/(K*m^2)  T_specify=off  T_priority=None  T=0 K  T_nominal_specify=off  T_nominal_value=1  T_nominal_unit=K  Q_specify=off  Q_priority=None  Q=0 W  Q_nominal_specify=off  Q_nominal_value=1  Q_nominal_unit=W
  Environment : FuelCell_lib/elements/Reservoir (FC)  constCond=true  p0=env_p MPa  T0=env_T degC  comp=FuelCell.enum.Composition.Mole  y0=[1-env_yO2-env_yH20; env_yO2; 0; env_yH20]  x0=[1; 0; 0; 0]  area=pi*anode_tube_D^2/4 m^2
      settings: InternalSimscapePortConfiguration="{\"Bottom\":[],\"Left\":[],\"Right\":[],\"Top\":[{\"id\":\"A\",\"label\":\"A\",\"type\":\"FuelCell.FuelCell\"}]}"
  Environment Temperature : fl_lib/Thermal/Thermal Sources/Temperature Source  temperature=env_T degC
  Max Area : fl_lib/Physical Signals/Functions/PS Gain  gain=pi*(anode_tube_D)^2/4 m^2
  PS-Simulink Converter : nesl_utility/PS-Simulink Converter  PhysicalDomain=network_engine_domain  SubClassName=ps_output  LeftPortType=input  RightPortType=output  PseudoPeriodic=off  Frequencies=[]  VectorFormat=inherit  Unit=inherit  AffineConversion=off
  Pipe (FC) : FuelCell_lib/elements/Pipe (FC)  length=1 m  area=pi*anode_tube_D^2/4 m^2  Dh=anode_tube_D m  extra_length=0.1 m  roughness=15e-6 m  Re_lam=2000  Re_tur=4000  shape_factor=64  Nu_lam=3.66  tau_c=1e-3 s  isCond=[0; 0; 0; 0]  volMeas=false  compMeas=FuelCell.enum.Composition.Mole  p0=env_p MPa  T0=env_T degC  comp=FuelCell.enum.Composition.Mole  y0=[0; 0; 1; 0]  x0=[1; 0; 0; 0]
      settings: InternalSimscapePortConfiguration="{\"Bottom\":[{\"id\":\"MIn\",\"label\":\"M_in\",\"type\":\"input\"},{\"id\":\"TIn\",\"label\":\"T_in\",\"type\":\"input\"}],\"Left\":[{\"id\":\"A\",\"label\":\"A\",\"type\":\"FuelCell.FuelCell\"},{\"id\":\"H\",\"label\":\"H\",\"type\":\"foundation.thermal.thermal\"}],\"Right\":[{\"id\":\"B\",\"label\":\"B\",\"type\":\"FuelCell.FuelCell\"}],\"Top\":[]}"
  Purge Valve : FuelCell_lib/elements/Local Restriction (FC)  const_area=false  restriction_area=0.001 m^2  min_area=pi*(1e-4*anode_tube_D)^2/4 m^2  max_area=pi*(0.5*anode_tube_D)^2/4 m^2  area=pi*anode_tube_D^2/4 m^2  Cd=0.64  B_lam=0.999
      settings: InternalSimscapePortConfiguration="{\"Bottom\":[],\"Left\":[{\"id\":\"AR\",\"label\":\"AR\",\"type\":\"input\"},{\"id\":\"A\",\"label\":\"A\",\"type\":\"FuelCell.FuelCell\"}],\"Right\":[{\"id\":\"B\",\"label\":\"B\",\"type\":\"FuelCell.FuelCell\"}],\"Top\":[]}"
  Purge_Active_Threshold : Sum  Inputs=+-
  Purge_Enable_Gate : Product
  Purge_N2_Error : Sum  Inputs=+-
  Purge_State_Memory : Memory
  Purge_State_Span : Product
  Purge_Threshold_Span : Sum  Inputs=+-
  Relay : Relay  OnSwitchValue=0  OffSwitchValue=-1e-9
  Simulink-PS Converter : nesl_utility/Simulink-PS Converter  PhysicalDomain=network_engine_domain  SubClassName=ps_input  LeftPortType=input  RightPortType=output  PseudoPeriodic=off  Frequencies=[]  NoiseDistribution=none  NoiseParameters=[]  Unit=1  AffineConversion=off  FilteringAndDerivatives=provide  SimscapeFilterOrder=1  InputFilterTimeConstant=0.001  UdotUserProvided=0
  Transfer Fcn : TransferFcn  Denominator=[1 5]
  yN2 : Selector  InputPortWidth=4  IndexOptions=Index vector (dialog)  Indices=1  OutputSizes=1
  A : PMIOPort  Side=Left
  tag scope: Purge=global, yN2=global
  wires:
  Transfer Fcn/1 -> Simulink-PS Converter/1
  yN2/1 -> [yN2], Purge_N2_Error/1
  PS-Simulink Converter/1 -> yN2/1
  [RouteA_CMD_anode_purge_on_n2_mole_fraction] -> Purge_Active_Threshold/1, Purge_Threshold_Span/1
  [RouteA_CMD_anode_purge_off_n2_mole_fraction] -> Purge_Threshold_Span/2
  Purge_State_Memory/1 -> Purge_State_Span/1
  Purge_Threshold_Span/1 -> Purge_State_Span/2
  Purge_State_Span/1 -> Purge_Active_Threshold/2
  Purge_Active_Threshold/1 -> Purge_N2_Error/2
  Purge_N2_Error/1 -> Relay/1
  Relay/1 -> Purge_Enable_Gate/1, Purge_State_Memory/1
  [RouteA_CMD_anode_purge_enable] -> Purge_Enable_Gate/2
  Purge_Enable_Gate/1 -> [Purge], Transfer Fcn/1
  connections:
  Pipe (FC)/LConn1 -- Composition and Humidity Sensor (FC)/LConn1 -- A/RConn1
  Simulink-PS Converter/RConn1 -- Max Area/LConn1
  Purge Valve/LConn1 -- Max Area/RConn1
  Convective Heat Transfer/LConn1 -- Pipe (FC)/LConn2
  Environment Temperature/LConn1 -- Convective Heat Transfer/RConn1
  Pipe (FC)/RConn1 -- Purge Valve/LConn2
  Environment/LConn1 -- Purge Valve/RConn1
  Composition and Humidity Sensor (FC)/RConn2 -- PS-Simulink Converter/LConn1

== system PEMFuelCellSystem_GasMixture_cEGR_RouteA_v2_v01/Anode_Hydrogen_BOP/Hydrogen Source ==
  Anode_Source_Conditioner : Subsystem
  Conditioner_to_Tank_Restriction : FuelCell_lib/elements/Local Restriction (FC)  const_area=true  restriction_area=0.95*pi*anode_tube_D^2/4 m^2  min_area=1e-10 m^2  max_area=0.99*pi*anode_tube_D^2/4 m^2  area=pi*anode_tube_D^2/4 m^2  Cd=0.8  B_lam=0.999
      settings: InternalSimscapePortConfiguration="{\"Bottom\":[],\"Left\":[{\"id\":\"A\",\"label\":\"A\",\"type\":\"FuelCell.FuelCell\"}],\"Right\":[{\"id\":\"B\",\"label\":\"B\",\"type\":\"FuelCell.FuelCell\"}],\"Top\":[]}"
  Constant1 : Constant  Value=0
  Fuel Tank : FuelCell_lib/elements/Constant Volume Chamber (FC)  V0=tank_V l  num_ports=foundation.enum.num_ports.one  area_A=0.01 m^2  area_B=0.01 m^2  area_C=0.01 m^2  area_D=0.01 m^2  cond_spec=FuelCell.enum.ChamberCondSpec.Enabled  tau_c=1 s  is_cond=[0; 0; 0; 0]  out_comp=FuelCell.enum.Composition.Mole  p0=tank_p MPa  T0=tank_T degC  comp=FuelCell.enum.Composition.Mole  y0=[1-tank_yH2; 0; tank_yH2; 0]  x0=[1; 0; 0; 0]
      settings: InternalSimscapePortConfiguration="{\"Bottom\":[{\"id\":\"H\",\"label\":\"H\",\"type\":\"foundation.thermal.thermal\"}],\"Left\":[{\"id\":\"MIn\",\"label\":\"MIn\",\"type\":\"input\"},{\"id\":\"TIn\",\"label\":\"TIn\",\"type\":\"input\"}],\"Right\":[{\"id\":\"pC\",\"label\":\"p\",\"type\":\"output\"},{\"id\":\"TC\",\"label\":\"T\",\"type\":\"output\"},{\"id\":\"yC_i\",\"label\":\"y_i\",\"type\":\"output\"}],\"Top\":[{\"id\":\"A\",\"label\":\"A\",\"type\":\"FuelCell.FuelCell\"}]}"
  Perfect Insulator : fl_lib/Thermal/Thermal Elements/Perfect Insulator  T_specify=off  T_priority=None  T=0 K  T_nominal_specify=off  T_nominal_value=1  T_nominal_unit=K
  Perfect Insulator1 : fl_lib/Thermal/Thermal Elements/Perfect Insulator  T_specify=off  T_priority=None  T=0 K  T_nominal_specify=off  T_nominal_value=1  T_nominal_unit=K
  Pipe (FC) : FuelCell_lib/elements/Pipe (FC)  length=1 m  area=pi*anode_tube_D^2/4 m^2  Dh=anode_tube_D m  extra_length=0.1 * 100 m  roughness=15e-6 m  Re_lam=2000  Re_tur=4000  shape_factor=64  Nu_lam=3.66  tau_c=1e-3 s  isCond=[0; 0; 0; 0]  volMeas=false  compMeas=FuelCell.enum.Composition.Mole  p0=env_p MPa  T0=env_T degC  comp=FuelCell.enum.Composition.Mole  y0=[0; 0; 1; 0]  x0=[1; 0; 0; 0]
      settings: InternalSimscapePortConfiguration="{\"Bottom\":[{\"id\":\"MIn\",\"label\":\"M_in\",\"type\":\"input\"},{\"id\":\"TIn\",\"label\":\"T_in\",\"type\":\"input\"}],\"Left\":[{\"id\":\"A\",\"label\":\"A\",\"type\":\"FuelCell.FuelCell\"},{\"id\":\"H\",\"label\":\"H\",\"type\":\"foundation.thermal.thermal\"}],\"Right\":[{\"id\":\"B\",\"label\":\"B\",\"type\":\"FuelCell.FuelCell\"}],\"Top\":[]}"
  Pressure-Reducing Valve : Subsystem  Tag=PublishSubsystem  mask(Pressure-Reducing Valve){D=anode_tube_D, r_min=1e-4, r_max=0.2, p_range=0.005}
      mask prompts: D "Connecting tube diameter (m)"; r_min "Min diameter ratio"; r_max "Max diameter ratio"; p_range "Pressure regulation range (MPa)"
      mask help: This subsystem models a pressure reducing valve that maintains a set pressure at port B. The valve is normally open. When the pressure is above the set pressure, it is fully closed.
  Simulink-PS Converter : nesl_utility/Simulink-PS Converter  PhysicalDomain=network_engine_domain  SubClassName=ps_input  LeftPortType=input  RightPortType=output  PseudoPeriodic=off  Frequencies=[]  NoiseDistribution=none  NoiseParameters=[]  Unit=MPa  AffineConversion=off  FilteringAndDerivatives=provide  SimscapeFilterOrder=1  InputFilterTimeConstant=0.001  UdotUserProvided=0
  Sum : Sum  Inputs=++|
  H2 : PMIOPort  Side=Right
  wires:
  [RouteA_CMD_anode_inlet_pressure_MPa_abs] -> Sum/1
  Constant1/1 -> Sum/2
  Sum/1 -> Simulink-PS Converter/1
  connections:
  Simulink-PS Converter/RConn1 -- Pressure-Reducing Valve/LConn2
  Perfect Insulator1/LConn1 -- Pipe (FC)/LConn2
  Pipe (FC)/RConn1 -- H2/RConn1
  Pressure-Reducing Valve/RConn1 -- Pipe (FC)/LConn1
  Perfect Insulator/LConn1 -- Fuel Tank/RConn4
  Fuel Tank/LConn3 -- Pressure-Reducing Valve/LConn1 -- Conditioner_to_Tank_Restriction/RConn1
  Anode_Source_Conditioner/RConn1 -- Conditioner_to_Tank_Restriction/LConn1

== system PEMFuelCellSystem_GasMixture_cEGR_RouteA_v2_v01/Anode_Hydrogen_BOP/Recirculation ==
  Constant Volume Chamber (FC) : FuelCell_lib/elements/Constant Volume Chamber (FC)  V0=0.05^3 m^3  num_ports=foundation.enum.num_ports.three  area_A=pi*anode_tube_D^2/4 m^2  area_B=pi*anode_tube_D^2/4 m^2  area_C=pi*anode_tube_D^2/4 m^2  area_D=0.01 m^2  cond_spec=FuelCell.enum.ChamberCondSpec.Enabled  tau_c=1e-3 s  is_cond=[0; 0; 0; 0]  out_comp=FuelCell.enum.Composition.Mole  p0=env_p MPa  T0=env_T degC  comp=FuelCell.enum.Composition.Mole  y0=[0; 0; 1; 0]  x0=[1; 0; 0; 0]
      settings: InternalSimscapePortConfiguration="{\"Bottom\":[{\"id\":\"H\",\"label\":\"H\",\"type\":\"foundation.thermal.thermal\"}],\"Left\":[{\"id\":\"MIn\",\"label\":\"MIn\",\"type\":\"input\"},{\"id\":\"TIn\",\"label\":\"TIn\",\"type\":\"input\"}],\"Right\":[{\"id\":\"pC\",\"label\":\"p\",\"type\":\"output\"},{\"id\":\"TC\",\"label\":\"T\",\"type\":\"output\"},{\"id\":\"yC_i\",\"label\":\"y_i\",\"type\":\"output\"}],\"Top\":[{\"id\":\"A\",\"label\":\"A\",\"type\":\"FuelCell.FuelCell\"},{\"id\":\"B\",\"label\":\"B\",\"type\":\"FuelCell.FuelCell\"},{\"id\":\"C\",\"label\":\"C\",\"type\":\"FuelCell.FuelCell\"}]}"
  Feedforward Control : Subsystem
  Mass Flow Rate Source (FC) : FuelCell_lib/sources/Mass Flow Rate Source (FC)  source_type=foundation.enum.constant_controlled.controlled  flow_rate=0 kg/s  power_spec=foundation.enum.power_spec.none  area_A=0.01 m^2  area_B=0.01 m^2  mdot_A_specify=off  mdot_A_priority=None  mdot_A=0.1 kg/s  mdot_A_nominal_specify=off  mdot_A_nominal_value=1  mdot_A_nominal_unit=kg/s  mdot_B_specify=off  mdot_B_priority=None  mdot_B=0.1 kg/s  mdot_B_nominal_specify=off  mdot_B_nominal_value=1  mdot_B_nominal_unit=kg/s  phi_A_specify=off  phi_A_priority=None  phi_A=0 J/s  phi_A_nominal_specify=off  phi_A_nominal_value=1  phi_A_nominal_unit=J/s  phi_B_specify=off  phi_B_priority=None  phi_B=0 J/s  phi_B_nominal_specify=off  phi_B_nominal_value=1  phi_B_nominal_unit=J/s  mdot_A_i_specify=off  mdot_A_i_priority=None  mdot_A_i=[0; 0; 0; 0] kg/s  mdot_A_i_nominal_specify=off  mdot_A_i_nominal_value=1  mdot_A_i_nominal_unit=kg/s  mdot_B_i_specify=off  mdot_B_i_priority=None  mdot_B_i=[0; 0; 0; 0] kg/s  mdot_B_i_nominal_specify=off  mdot_B_i_nominal_value=1  mdot_B_i_nominal_unit=kg/s
      settings: InternalSimscapePortConfiguration="{\"Bottom\":[],\"Left\":[{\"id\":\"M\",\"label\":\"M\",\"type\":\"input\"},{\"id\":\"A\",\"label\":\"A\",\"type\":\"FuelCell.FuelCell\"}],\"Right\":[{\"id\":\"B\",\"label\":\"B\",\"type\":\"FuelCell.FuelCell\"}],\"Top\":[]}"
  Max Flow : fl_lib/Physical Signals/Functions/PS Gain  gain=0.01 kg/s
  Perfect Insulator : fl_lib/Thermal/Thermal Elements/Perfect Insulator  T_specify=off  T_priority=None  T=0 K  T_nominal_specify=off  T_nominal_value=1  T_nominal_unit=K
  Simulink-PS Converter : nesl_utility/Simulink-PS Converter  PhysicalDomain=network_engine_domain  SubClassName=ps_input  LeftPortType=input  RightPortType=output  PseudoPeriodic=off  Frequencies=[]  NoiseDistribution=none  NoiseParameters=[]  Unit=1  AffineConversion=off  FilteringAndDerivatives=provide  SimscapeFilterOrder=1  InputFilterTimeConstant=0.001  UdotUserProvided=0
  A : PMIOPort  Side=Left
  B : PMIOPort  Port=2  Side=Right
  R : PMIOPort  Port=3  Side=Right
  wires:
  [i_stack] -> Feedforward Control/1(i)
  Feedforward Control/1(cmd) -> Simulink-PS Converter/1
  connections:
  Max Flow/RConn1 -- Mass Flow Rate Source (FC)/LConn1
  Simulink-PS Converter/RConn1 -- Max Flow/LConn1
  R/RConn1 -- Mass Flow Rate Source (FC)/LConn2
  Perfect Insulator/LConn1 -- Constant Volume Chamber (FC)/RConn4
  Constant Volume Chamber (FC)/LConn4 -- Mass Flow Rate Source (FC)/RConn1
  A/RConn1 -- Constant Volume Chamber (FC)/LConn3
  B/RConn1 -- Constant Volume Chamber (FC)/LConn5

== system PEMFuelCellSystem_GasMixture_cEGR_RouteA_v2_v01/Anode_Hydrogen_BOP/Subsystem ==
  N2 : Outport
  Purge : Outport  Port=2
  wires:
  [yN2] -> N2/1  "N2 molar fraction"
  [Purge] -> Purge/1  "Purge valve enabled"
